simulink model "SolutionP3"  (R2018b)
settings: Solver=VariableStepAuto  StartTime=0.0  StopTime=tmax  MaxStep=0.1  RelTol=1e-3
values from neighbouring files (symbols this model uses):
  A = sys.A    [SolutionP1.m]    (also in SolutionP22.m = [0, -a0;1, -a1]; SolutionP2KalmanFilter.m = [0 -a2; SolutionP31.m = [0, -a0;1, -a1])
  a0 = 1    [SolutionP1.m]    (also in SolutionP22.m; SolutionP31.m)
  a1 = 0.5    [SolutionP1.m]    (also in SolutionP22.m = 0.2; SolutionP2KalmanFilter.m = -1.5; SolutionP31.m = 0.2)
  B = [b0; 0]    [SolutionP22.m]    (also in SolutionP2KalmanFilter.m = [0 b0]'; SolutionP31.m)
  b0 = 1    [SolutionP1.m]    (also in SolutionP22.m; SolutionP2KalmanFilter.m = 0.9; SolutionP31.m)
  C = [0 1]    [SolutionP22.m]    (also in SolutionP2KalmanFilter.m = [0 1]'; SolutionP31.m)
  K = P*C/(rv + C'*P*C)    [SolutionP2KalmanFilter.m]    (also in SolutionP31.m = 1*[1,.1])
  L = [.2; .1]    [SolutionP22.m]    (also in SolutionP2KalmanFilter.m = 2; SolutionP31.m)
settings Model: Creator=raphael  LastModifiedBy=raphael

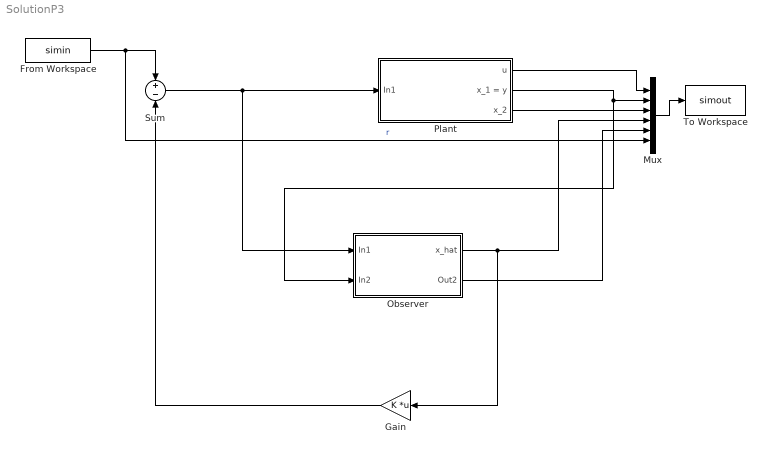
== system SolutionP3 ==
  From Workspace : FromWorkspace  VariableName=simin  SampleTime=0
  Gain : Gain  Gain=K  Multiplication=Matrix(K*u) (u vector)
  Mux : Mux  Inputs=6
  Observer : Subsystem
  Plant : Subsystem
  Sum : Sum  Inputs=+-
  To Workspace : ToWorkspace  VariableName=simout  SaveFormat=Timeseries  SampleTime=-1
  wires:
  Mux/1 -> To Workspace/1
  Plant/1(u) -> Mux/1
  Plant/2(x_1 = y) -> Observer/2(In2), Mux/2
  Plant/3(x_2) -> Mux/3
  Observer/1(x_hat) -> Gain/1, Mux/4
  Observer/2(Out2) -> Mux/5
  From Workspace/1 -> Mux/6, Sum/1  "r"
  Sum/1 -> Observer/1(In1), Plant/1(In1)
  Gain/1 -> Sum/2

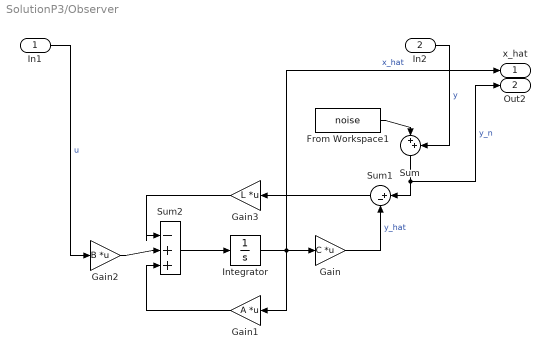
== system SolutionP3/Observer ==
  In1 : Inport
  In2 : Inport  Port=2
  From Workspace1 : FromWorkspace  VariableName=noise  SampleTime=0
  Gain : Gain  Gain=C  Multiplication=Matrix(K*u) (u vector)
  Gain1 : Gain  Gain=A  Multiplication=Matrix(K*u) (u vector)
  Gain2 : Gain  Gain=B  Multiplication=Matrix(K*u) (u vector)
  Gain3 : Gain  Gain=L  Multiplication=Matrix(K*u)
  Integrator : Integrator
  Sum : Sum  Inputs=|++
  Sum1 : Sum  Inputs=|+-
  Sum2 : Sum  Inputs=|-++
  x_hat : Outport
  Out2 : Outport  Port=2
  wires:
  In1/1 -> Gain2/1  "u"
  Sum2/1 -> Integrator/1
  Gain2/1 -> Sum2/2
  From Workspace1/1 -> Sum/1
  Gain3/1 -> Sum2/1
  Gain1/1 -> Sum2/3
  Gain/1 -> Sum1/2  "y_hat"
  Sum/1 -> Out2/1, Sum1/1  "y_n"
  Sum1/1 -> Gain3/1
  In2/1 -> Sum/2  "y"
  Integrator/1 -> Gain1/1, x_hat/1, Gain/1  "x_hat"

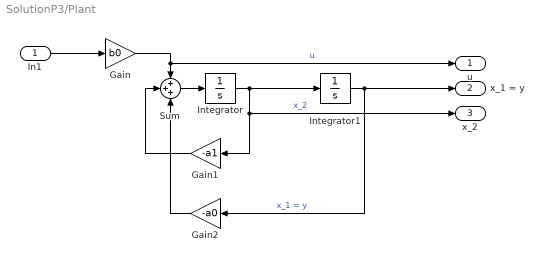
== system SolutionP3/Plant ==
  In1 : Inport
  Gain : Gain  Gain=b0
  Gain1 : Gain  Gain=-a1
  Gain2 : Gain  Gain=-a0
  Integrator : Integrator
  Integrator1 : Integrator
  Sum : Sum  Inputs=+++
  u : Outport
  x_1 = y : Outport  Port=2
  x_2 : Outport  Port=3
  wires:
  Gain2/1 -> Sum/3
  Sum/1 -> Integrator/1
  Integrator/1 -> Integrator1/1, Gain1/1, x_2/1  "x_2"
  In1/1 -> Gain/1
  Integrator1/1 -> x_1 = y/1, Gain2/1  "x_1 = y"
  Gain1/1 -> Sum/2
  Gain/1 -> u/1, Sum/1  "u"
